simulink model "00SimulinkExample"  (R2022b)
settings: Solver=FixedStepAuto  StartTime=0.0  StopTime=10.0  FixedStep=1e-06  RelTol=1e-3
model workspace (MAT data in the model file):
  Sig = Simulink.Signal
  Sig.DataType = 'auto'
  Sig.Dimensions = -1
  Sig.DimensionsMode = 'auto'
  Sig.Complexity = 'auto'
  Sig.SampleTime = -1
  Sig.SamplingMode = 'auto'
settings Model: DataDictionary=BusSystem.sldd  Creator=Finn  LastModifiedBy=cao2851
settings SolverCC: AlgebraicLoopSolver=TrustRegion
settings DebuggingCC: UnconnectedInputMsg=warning  UnconnectedOutputMsg=warning  UnconnectedLineMsg=warning  SFMachineParentedDataDiag=warning
settings HardwareCC: TargetBitPerLong=64  TargetBitPerPointer=64  TargetBitPerSizeT=64  TargetBitPerPtrDiffT=64  TargetLongLongMode=on  TargetIntDivRoundTo=Zero  TargetEndianess=LittleEndian  TargetWordSize=64  TargetHWDeviceType=MATLAB Host  ProdEqTarget=off
settings ModelReferenceCC: EnableRefExpFcnMdlSchedulingChecks=on
settings RTWCC: Description=S-Function Target  SystemTargetFile=rtwsfcn.tlc  TemplateMakefile=rtwsfcn_default_tmf  RetainRTWFile=on  DLArmComputeVersion=19.05
settings STFCustomTargetCC: TargetLangStandard=C99 (ISO)  ModelReferenceCompliant=off  CompOptLevelCompliant=on  MATLABClassNameForMDSCustomization=Simulink.SoftwareTarget.TargetSpecificTriggerConfigurationBase  GRTInterface=on  SystemTargetFile=rtwsfcn.tlc

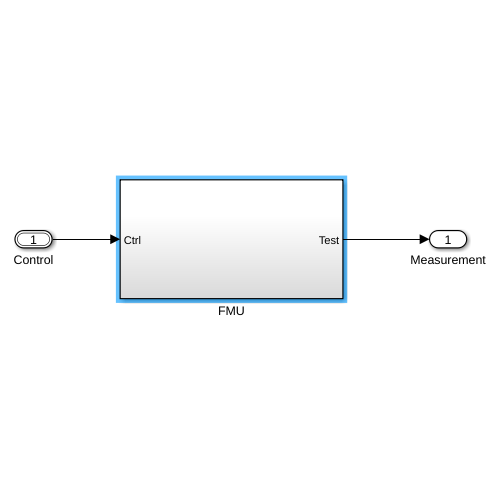
[thumbnail: Simulink's stored preview of the top-level diagram]
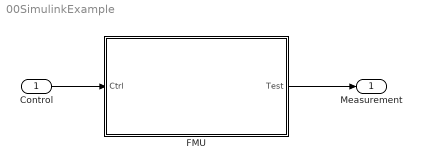
== system 00SimulinkExample ==
  Control : Inport  OutDataTypeStr=Bus: bus3
  FMU : Subsystem
  Measurement : Outport
  wires:
  Control/1 -> FMU/1(Ctrl)
  FMU/1(Test) -> Measurement/1

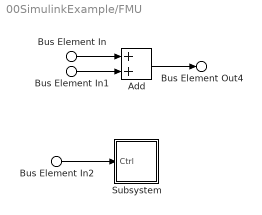
== system 00SimulinkExample/FMU ==
  Bus Element In : Inport  PortName=Ctrl  Element=Sum1
  Bus Element In1 : Inport  PortName=Ctrl  Element=Sum2
  Bus Element In2 : Inport  PortName=Ctrl  Element=Terminated
  Add : Sum
  Subsystem : Subsystem
  Bus Element Out4 : Outport  PortName=Test  Element=SumOut
  wires:
  Bus Element In/1 -> Add/1
  Bus Element In1/1 -> Add/2
  Add/1 -> Bus Element Out4/1
  Bus Element In2/1 -> Subsystem/1(Ctrl)

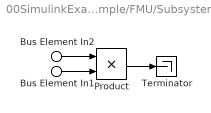
== system 00SimulinkExample/FMU/Subsystem ==
  Bus Element In1 : Inport  PortName=Ctrl  Element=Signal2
  Bus Element In2 : Inport  PortName=Ctrl  Element=Signal1
  Product : Product
  Terminator : Terminator
  wires:
  Bus Element In1/1 -> Product/2
  Bus Element In2/1 -> Product/1
  Product/1 -> Terminator/1
